simulink model "Basic_models_vfinal"  (R2019b)
settings: Solver=ode4  StartTime=0.0  StopTime=0.2  FixedStep=1e-5  MaxStep=1e-4  RelTol=1e-5
undefined symbols (not defined in the file or in its folder): C, L, R, R1
libraries: powerlib x82, powerlib_meascontrol x25
settings Model: Creator=eprie  LastModifiedBy=Edu Prieto

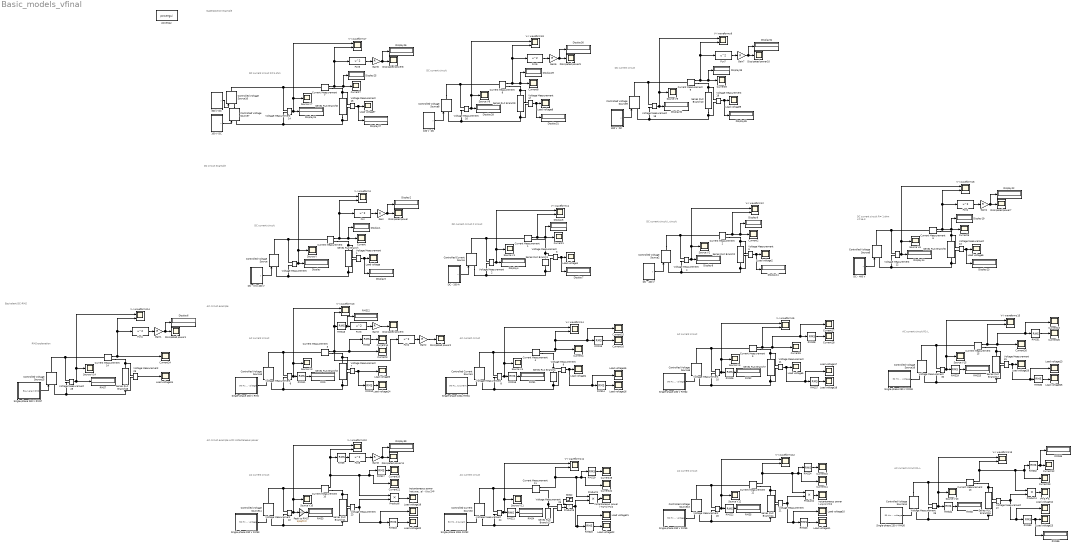
== system Basic_models_vfinal ==
  note: DC circuit example
  note: DC current circuit
  note: DC current circuit
      | C circuit
  note: DC current circuit
      | L circuit
  note: AC current circuit
  note: AC current circuit
  note: AC current circuit
  note: DC current circuit
      | R= 1 ohm L=1e-3
  note: DC current circuit
      | R=1 ohm
  note: DC current circuit
  note: DC current circuit
  note: Superposition example
  note: AC circuit example
  note: AC current circuit
  note: AC current circuit
  note: AC current circuit
  note: AC circuit example
      | with instantaneous power
  note: AC current circuit
      | R1-L
  note: RMS explanation
  note: Equivalent DC-RMS
  note: AC current circuit
      | R1-L
  "100 V  DC " : Subsystem
  100 V DC : Subsystem
  300 V  DC : Subsystem
  300 V DC : Subsystem
  Controlled Current Source : powerlib/Electrical Sources/Controlled Current Source  Initialize=on  Source_Type=AC  Amplitude=0  Phase=0  Frequency=0  Measurements=None
      settings: SourceProductName=Simscape Electrical
  Controlled Current Source1 : powerlib/Electrical Sources/Controlled Current Source  Initialize=off  Source_Type=AC  Amplitude=0  Phase=0  Frequency=0  Measurements=None
      settings: SourceProductName=Simscape Electrical
  Controlled Current Source2 : powerlib/Electrical Sources/Controlled Current Source  Initialize=off  Source_Type=AC  Amplitude=0  Phase=0  Frequency=0  Measurements=None
      settings: SourceProductName=Simscape Electrical
  Controlled Voltage Source{,2..3,5..11,13..16} (14 alike) : powerlib/Electrical Sources/Controlled Voltage Source  Initialize=on  Source_Type=AC  Amplitude=0  Phase=0  Frequency=0  Measurements=None
      settings: SourceProductName=Simscape Electrical
  Current{,1..26} (27 alike) : Scope
  Current Measurement{,1..15} (16 alike) : powerlib/Measurements/Current Measurement  PhasorSimulation=off  OutputType=Complex  PSBequivalent=0
      settings: SourceProductName=Simscape Electrical
  DC - 0 to 400 V : Subsystem
  DC - 200 A : Subsystem
  DC - 400 V : Subsystem
  "DC - 400 V  " : Subsystem
  Display{,1..9,11,14,19,22..35,39} (28 alike) : Display
  Dissipated power{,1..3,7..11} (9 alike) : Scope
  Fcn{,1..8} (9 alike) : Fcn  Expr=u^2
  Gain{,1..8} (9 alike) : Gain  Gain=R
  "Instantaneous power (+S/-S) P=0 " : Scope
  "Instantaneous power (+S/-S) P=0 " : Scope
  Instantaneous power (not average) - 0 to 2*P : Scope
  Load voltage{,1..26} (27 alike) : Scope
  P+S P-S : Scope
  Peak to RMS7 : Gain  Gain=1/sqrt(2)
  Product{1..2,4..6} (5 alike) : Product
  RMS{,1..7,12,25,35..36} (12 alike) : Display
  RMS{8..11,13..24,26..34} (25 alike) : powerlib_meascontrol/Measurements/RMS  TrueRMS=on  Freq=50  RMSInit=120  Ts=0
      settings: SourceProductName=Simscape Electrical
  Series RLC Branch{,3,8..11,16} (7 alike) : powerlib/Elements/Series RLC Branch  LConnTagsString=__new0  RConnTagsString=__new0  BranchType=R  Resistance=R  Inductance=1e-3  SetiL0=off  InitialCurrent=0  Capacitance=1e-6  Setx0=off  InitialVoltage=0  Measurements=None
      settings: SourceProductName=Simscape Electrical
  Series RLC Branch1 : powerlib/Elements/Series RLC Branch  LConnTagsString=__new0  RConnTagsString=__new0  BranchType=C  Resistance=R  Inductance=1e-3  SetiL0=off  InitialCurrent=0  Capacitance=C  Setx0=off  InitialVoltage=0  Measurements=None
      settings: SourceProductName=Simscape Electrical
  Series RLC Branch12 : powerlib/Elements/Series RLC Branch  LConnTagsString=__new0  RConnTagsString=__new0  BranchType=C  Resistance=1e-4  Inductance=1e-3  SetiL0=off  InitialCurrent=0  Capacitance=C  Setx0=off  InitialVoltage=400/sqrt(3)*sqrt(2)  Measurements=None
      settings: SourceProductName=Simscape Electrical
  Series RLC Branch14 : powerlib/Elements/Series RLC Branch  LConnTagsString=__new0  RConnTagsString=__new0  BranchType=L  Resistance=R  Inductance=L  SetiL0=off  InitialCurrent=0  Capacitance=1e-6  Setx0=off  InitialVoltage=0  Measurements=None
      settings: SourceProductName=Simscape Electrical
  Series RLC Branch15 : powerlib/Elements/Series RLC Branch  LConnTagsString=__new0  RConnTagsString=__new0  BranchType=RL  Resistance=R1  Inductance=L  SetiL0=off  InitialCurrent=0  Capacitance=1e-6  Setx0=off  InitialVoltage=0  Measurements=None
      settings: SourceProductName=Simscape Electrical
  Series RLC Branch17 : powerlib/Elements/Series RLC Branch  LConnTagsString=__new0  RConnTagsString=__new0  BranchType=RL  Resistance=R1  Inductance=L  SetiL0=off  InitialCurrent=0  Capacitance=1e-6  Setx0=off  InitialVoltage=0  Measurements=None
      settings: SourceProductName=Simscape Electrical
  Series RLC Branch2 : powerlib/Elements/Series RLC Branch  LConnTagsString=__new0  RConnTagsString=__new0  BranchType=L  Resistance=0.00001  Inductance=L  SetiL0=off  InitialCurrent=0  Capacitance=C  Setx0=off  InitialVoltage=0  Measurements=None
      settings: SourceProductName=Simscape Electrical
  Series RLC Branch4 : powerlib/Elements/Series RLC Branch  LConnTagsString=__new0  RConnTagsString=__new0  BranchType=C  Resistance=1e-4  Inductance=1e-3  SetiL0=off  InitialCurrent=0  Capacitance=C  Setx0=off  InitialVoltage=400/sqrt(3)*sqrt(2)  Measurements=None
      settings: SourceProductName=Simscape Electrical
  Series RLC Branch5 : powerlib/Elements/Series RLC Branch  LConnTagsString=__new0  RConnTagsString=__new0  BranchType=RL  Resistance=R  Inductance=L  SetiL0=off  InitialCurrent=0  Capacitance=1e-6  Setx0=off  InitialVoltage=0  Measurements=None
      settings: SourceProductName=Simscape Electrical
  Series RLC Branch7 : powerlib/Elements/Series RLC Branch  LConnTagsString=__new0  RConnTagsString=__new0  BranchType=L  Resistance=R  Inductance=L  SetiL0=off  InitialCurrent=0  Capacitance=1e-6  Setx0=off  InitialVoltage=0  Measurements=None
      settings: SourceProductName=Simscape Electrical
  Single-phase 100A RMS1 : Subsystem
  Single-phase 100A RMS2 : Subsystem
  Single-phase 230 V RMS : Subsystem
  Single-phase 230 V RMS2 : Subsystem
  Single-phase 230 V RMS3 : Subsystem
  Single-phase 230 V RMS5 : Subsystem
  Single-phase 230 V RMS6 : Subsystem
  Single-phase 230 V RMS7 : Subsystem
  Single-phase 230 V RMS8 : Subsystem
  Source V{,1..15} (16 alike) : Scope
  Step2 : Step  Time=0.01  SampleTime=0
  V-I waveforms{,1..15} (16 alike) : Scope  NumInputPorts=2
  Voltage Measurement{,1..31} (32 alike) : powerlib/Measurements/Voltage Measurement  PhasorSimulation=off  OutputType=Complex  PSBequivalent=0
      settings: SourceProductName=Simscape Electrical
  powergui : powerlib/powergui  Priority=1  SimulationMode=Discrete  SampleTime=1e-5  frequency=60  Iterations=50  frequencyindice=0  Pbase=100e6  ErrMax=1e-4  UnitsV=kV  UnitsW=MW  buscounter=0  FunctionMessages=off  echomessages=off  EnableUseOfTLC=off  CurrentSourceSwitches=off  DisableSnubberDevices=off  DisableRonSwitches=off  DisableVfSwitches=off  DisplayEquations=off  AutomaticDiscreteSolvers=off  SolverType=Tustin/Backward Euler (TBE)  Interpol=off  ExternalGateDelay=off  methode=off  Ts=100  x0status=blocks  SPID=on  SwTol=0  HookPort=off  NonlinearTolerance=1e-4  nMaxIteration=100  ContinueOnMaxIteration=off  RestoreLinks=warning  ResistiveCurrentMeasurement=off  Frange=[0:2:500]  Ylog=off  Xlog=on  ShowGrid=off  save=off  variable=ZData  structure=0  ZoomFFT=off  StartTime=0.0  cycles=1  DisplayStyle=1  fundamental=60  FreqAxis=off  MaxFrequency=1000  frequencyindicesteady=1  RmsSteady=1  display=off
      settings: SourceProductName=Simscape Electrical
  wires:
  Current Measurement/1 -> Current/1, Display1/1, V-I waveforms/2, Fcn/1
  DC - 0 to 400 V/1(v) -> Controlled Voltage Source/1
  Fcn/1 -> Gain/1
  Gain/1 -> Display2/1, Dissipated power/1
  Voltage Measurement/1 -> V-I waveforms/1, Source V/1, Display/1
  Voltage Measurement1/1 -> Display3/1, Load voltage/1
  Voltage Measurement3/1 -> Load voltage1/1, Display7/1
  Voltage Measurement2/1 -> Display4/1, Source V1/1, V-I waveforms1/1
  DC - 200 A/1(v) -> Controlled Current Source/1
  Current Measurement1/1 -> V-I waveforms1/2, Display5/1, Current1/1
  Current Measurement2/1 -> Current2/1, Display9/1, V-I waveforms2/2
  DC - 400 V/1(v) -> Controlled Voltage Source2/1
  Voltage Measurement4/1 -> V-I waveforms2/1, Source V2/1, Display8/1
  Voltage Measurement5/1 -> Display11/1, Load voltage2/1
  Voltage Measurement6/1 -> Source V3/1, V-I waveforms3/1, RMS11/1
  Gain3/1 -> Dissipated power3/1
  Fcn3/1 -> Gain3/1
  Single-phase 230 V RMS/1(50 Hz AC voltage) -> Controlled Voltage Source3/1
  RMS11/1 -> RMS/1
  RMS13/1 -> RMS12/1, Fcn3/1
  Voltage Measurement7/1 -> RMS10/1, Load voltage3/1
  Current Measurement3/1 -> RMS13/1, V-I waveforms3/2, Fcn2/1, RMS8/1, Current3/1
  Current Measurement4/1 -> V-I waveforms4/2, Current15/1, RMS15/1, Current4/1
  Voltage Measurement9/1 -> Load voltage15/1, RMS14/1, Load voltage4/1
  RMS16/1 -> RMS1/1
  Single-phase 100A RMS1/1(50 Hz AC current) -> Controlled Current Source1/1
  Voltage Measurement8/1 -> V-I waveforms4/1, Source V4/1, RMS16/1
  Voltage Measurement10/1 -> Source V5/1, V-I waveforms5/1, RMS26/1
  Single-phase 230 V RMS2/1(50 Hz AC voltage) -> Controlled Voltage Source5/1
  RMS26/1 -> RMS2/1
  Voltage Measurement11/1 -> RMS27/1, Load voltage17/1, Load voltage5/1
  Current Measurement5/1 -> V-I waveforms5/2, RMS28/1, Current17/1, Current5/1
  RMS10/1 -> Load voltage14/1
  RMS15/1 -> Current16/1
  RMS14/1 -> Load voltage16/1
  RMS28/1 -> Current18/1
  RMS27/1 -> Load voltage18/1
  Voltage Measurement13/1 -> Load voltage6/1, Display23/1
  Voltage Measurement12/1 -> Display14/1, Source V6/1, V-I waveforms6/1
  Gain4/1 -> Dissipated power7/1, Display22/1
  Fcn4/1 -> Gain4/1
  "DC - 400 V  "/1(v) -> Controlled Voltage Source6/1
  Current Measurement6/1 -> Fcn4/1, V-I waveforms6/2, Display19/1, Current6/1
  Voltage Measurement15/1 -> Load voltage7/1, Display27/1
  Voltage Measurement14/1 -> Display24/1, Source V7/1, V-I waveforms7/1
  Gain5/1 -> Dissipated power8/1, Display26/1
  Fcn5/1 -> Gain5/1
  100 V DC/1(v) -> Controlled Voltage Source7/1
  Current Measurement7/1 -> Fcn5/1, V-I waveforms7/2, Display25/1, Current7/1
  Current Measurement8/1 -> Current8/1, Display29/1, V-I waveforms8/2, Fcn6/1
  "100 V  DC "/1(v) -> Controlled Voltage Source8/1
  Fcn6/1 -> Gain6/1
  Gain6/1 -> Display30/1, Dissipated power9/1
  Voltage Measurement16/1 -> V-I waveforms8/1, Source V8/1, Display28/1
  Voltage Measurement17/1 -> Display31/1, Load voltage8/1
  Voltage Measurement19/1 -> Load voltage9/1, Display35/1
  Voltage Measurement18/1 -> Display32/1, Source V9/1, V-I waveforms9/1
  Gain7/1 -> Dissipated power10/1, Display34/1
  Fcn7/1 -> Gain7/1
  300 V  DC/1(v) -> Controlled Voltage Source9/1
  Current Measurement9/1 -> Fcn7/1, V-I waveforms9/2, Display33/1, Current9/1
  300 V DC/1(v) -> Controlled Voltage Source10/1
  RMS17/1 -> Current20/1
  Product6/1 -> Instantaneous power (not average) - 0 to 2*P/1
  RMS22/1 -> RMS5/1
  Single-phase 230 V RMS5/1(50 Hz AC voltage) -> Controlled Voltage Source13/1
  Voltage Measurement20/1 -> V-I waveforms12/1, Source V12/1, RMS22/1
  Voltage Measurement24/1 -> Source V11/1, V-I waveforms11/1, RMS21/1
  Single-phase 100A RMS2/1(50 Hz AC current) -> Controlled Current Source2/1
  RMS21/1 -> RMS4/1
  RMS9/1 -> Fcn8/1
  Peak to RMS7/1 -> RMS3/1
  Single-phase 230 V RMS3/1(50 Hz AC voltage) -> Controlled Voltage Source11/1
  Fcn8/1 -> Gain8/1
  Gain8/1 -> Display39/1, Dissipated power11/1
  Voltage Measurement22/1 -> V-I waveforms10/1, Source V10/1, Peak to RMS7/1
  Voltage Measurement26/1 -> RMS34/1, Source V13/1, V-I waveforms13/1
  Single-phase 230 V RMS6/1(50 Hz AC voltage) -> Controlled Voltage Source14/1
  RMS34/1 -> RMS6/1
  RMS8/1 -> Current14/1
  RMS18/1 -> Load voltage20/1
  Product5/1 -> Product1/2, RMS20/1, Load voltage21/1
  RMS20/1 -> Load voltage22/1
  Current Measurement11/1 -> Product1/1, Current22/1, RMS19/1, V-I waveforms11/2
  Product1/1 -> "Instantaneous power (+S/-S) P=0 "/1
  RMS19/1 -> Current19/1
  RMS24/1 -> Current10/1
  Product2/1 -> "Instantaneous power (+S/-S) P=0 "/1
  Current Measurement12/1 -> Current11/1, RMS24/1, Product2/1, V-I waveforms12/2
  RMS23/1 -> Load voltage11/1
  Voltage Measurement21/1 -> Product2/2, RMS23/1, Load voltage10/1
  Voltage Measurement27/1 -> Product4/2, RMS33/1, Load voltage12/1
  RMS33/1 -> RMS36/1, Load voltage23/1
  Current Measurement13/1 -> V-I waveforms13/2, Product4/1, RMS32/1, Current23/1
  Product4/1 -> P+S P-S/1
  RMS32/1 -> RMS35/1, Current12/1
  Current Measurement10/1 -> Product6/1, Current21/1, RMS17/1, RMS9/1, V-I waveforms10/2
  Voltage Measurement23/1 -> Product6/2, RMS18/1, Load voltage19/1
  Step2/1 -> Product5/1
  Voltage Measurement25/1 -> Product5/2
  Voltage Measurement29/1 -> Load voltage24/1
  Current Measurement14/1 -> Current24/1, Fcn1/1, V-I waveforms14/2
  Voltage Measurement28/1 -> RMS7/1, V-I waveforms14/1, Source V14/1
  Single-phase 230 V RMS7/1(Equivalent RMS) -> Controlled Voltage Source15/1
  Fcn1/1 -> Gain1/1
  Gain1/1 -> Display6/1, Dissipated power1/1
  RMS30/1 -> Load voltage25/1
  RMS31/1 -> Current25/1
  Current Measurement15/1 -> Current26/1, RMS31/1, Current13/1, V-I waveforms15/2
  Voltage Measurement31/1 -> Load voltage26/1, Load voltage13/1, RMS30/1
  RMS29/1 -> RMS25/1
  Single-phase 230 V RMS8/1(50 Hz AC voltage) -> Controlled Voltage Source16/1
  Voltage Measurement30/1 -> V-I waveforms15/1, Source V15/1, RMS29/1
  Fcn2/1 -> Gain2/1
  Gain2/1 -> Dissipated power2/1
  connections:
  Current Measurement/LConn1 -- Voltage Measurement/LConn1 -- Controlled Voltage Source/RConn1
  Current Measurement/RConn1 -- Series RLC Branch/LConn1 -- Voltage Measurement1/LConn1
  Series RLC Branch/RConn1 -- Voltage Measurement/LConn2 -- Controlled Voltage Source/LConn1 -- Voltage Measurement1/LConn2
  Voltage Measurement2/LConn1 -- Controlled Current Source/RConn1 -- Current Measurement1/LConn1
  Series RLC Branch1/RConn1 -- Voltage Measurement3/LConn2 -- Controlled Current Source/LConn1 -- Voltage Measurement2/LConn2
  Controlled Voltage Source2/RConn1 -- Voltage Measurement4/LConn1 -- Current Measurement2/LConn1
  Voltage Measurement5/LConn1 -- Current Measurement2/RConn1 -- Series RLC Branch2/LConn1
  Voltage Measurement5/LConn2 -- Series RLC Branch2/RConn1 -- Voltage Measurement4/LConn2 -- Controlled Voltage Source2/LConn1
  Voltage Measurement6/LConn1 -- Current Measurement3/LConn1 -- Controlled Voltage Source3/RConn1
  Current Measurement3/RConn1 -- Voltage Measurement7/LConn1 -- Series RLC Branch3/LConn1
  Series RLC Branch3/RConn1 -- Voltage Measurement7/LConn2 -- Voltage Measurement6/LConn2 -- Controlled Voltage Source3/LConn1
  Voltage Measurement8/LConn1 -- Controlled Current Source1/RConn1 -- Current Measurement4/LConn1
  Controlled Current Source1/LConn1 -- Voltage Measurement8/LConn2 -- Series RLC Branch4/RConn1 -- Voltage Measurement9/LConn2
  Voltage Measurement10/LConn1 -- Current Measurement5/LConn1 -- Controlled Voltage Source5/RConn1
  Current Measurement5/RConn1 -- Voltage Measurement11/LConn1 -- Series RLC Branch7/LConn1
  Voltage Measurement10/LConn2 -- Series RLC Branch7/RConn1 -- Voltage Measurement11/LConn2 -- Controlled Voltage Source5/LConn1
  Voltage Measurement9/LConn1 -- Current Measurement4/RConn1 -- Series RLC Branch4/LConn1
  Current Measurement6/LConn1 -- Voltage Measurement12/LConn1 -- Controlled Voltage Source6/RConn1
  Current Measurement6/RConn1 -- Voltage Measurement13/LConn1 -- Series RLC Branch5/LConn1
  Series RLC Branch5/RConn1 -- Voltage Measurement13/LConn2 -- Voltage Measurement12/LConn2 -- Controlled Voltage Source6/LConn1
  Current Measurement7/LConn1 -- Controlled Voltage Source10/RConn1 -- Voltage Measurement14/LConn1
  Current Measurement7/RConn1 -- Voltage Measurement15/LConn1 -- Series RLC Branch8/LConn1
  Series RLC Branch8/RConn1 -- Voltage Measurement15/LConn2 -- Voltage Measurement14/LConn2 -- Controlled Voltage Source7/LConn1
  Controlled Voltage Source8/RConn1 -- Current Measurement8/LConn1 -- Voltage Measurement16/LConn1
  Voltage Measurement17/LConn1 -- Current Measurement8/RConn1 -- Series RLC Branch9/LConn1
  Controlled Voltage Source8/LConn1 -- Series RLC Branch9/RConn1 -- Voltage Measurement17/LConn2 -- Voltage Measurement16/LConn2
  Current Measurement9/LConn1 -- Voltage Measurement18/LConn1 -- Controlled Voltage Source9/RConn1
  Current Measurement9/RConn1 -- Voltage Measurement19/LConn1 -- Series RLC Branch10/LConn1
  Series RLC Branch10/RConn1 -- Voltage Measurement18/LConn2 -- Controlled Voltage Source9/LConn1 -- Voltage Measurement19/LConn2
  Controlled Voltage Source10/LConn1 -- Controlled Voltage Source7/RConn1
  Voltage Measurement22/LConn1 -- Controlled Voltage Source11/RConn1 -- Current Measurement10/LConn1
  Current Measurement10/RConn1 -- Series RLC Branch11/LConn1 -- Voltage Measurement23/LConn1
  Series RLC Branch11/RConn1 -- Controlled Voltage Source11/LConn1 -- Voltage Measurement22/LConn2 -- Voltage Measurement23/LConn2
  Voltage Measurement24/LConn1 -- Controlled Current Source2/RConn1 -- Current Measurement11/LConn1
  Voltage Measurement24/LConn2 -- Controlled Current Source2/LConn1 -- Series RLC Branch12/RConn1 -- Voltage Measurement25/LConn2
  Voltage Measurement20/LConn1 -- Controlled Voltage Source13/RConn1 -- Current Measurement12/LConn1
  Current Measurement12/RConn1 -- Series RLC Branch14/LConn1 -- Voltage Measurement21/LConn1
  Voltage Measurement20/LConn2 -- Controlled Voltage Source13/LConn1 -- Voltage Measurement21/LConn2 -- Series RLC Branch14/RConn1
  Voltage Measurement25/LConn1 -- Current Measurement11/RConn1 -- Series RLC Branch12/LConn1
  Controlled Voltage Source14/RConn1 -- Voltage Measurement26/LConn1 -- Current Measurement13/LConn1
  Series RLC Branch15/LConn1 -- Current Measurement13/RConn1 -- Voltage Measurement27/LConn1
  Voltage Measurement27/LConn2 -- Voltage Measurement26/LConn2 -- Controlled Voltage Source14/LConn1 -- Series RLC Branch15/RConn1
  Voltage Measurement28/LConn1 -- Controlled Voltage Source15/RConn1 -- Current Measurement14/LConn1
  Current Measurement14/RConn1 -- Series RLC Branch16/LConn1 -- Voltage Measurement29/LConn1
  Series RLC Branch16/RConn1 -- Controlled Voltage Source15/LConn1 -- Voltage Measurement28/LConn2 -- Voltage Measurement29/LConn2
  Voltage Measurement30/LConn1 -- Controlled Voltage Source16/RConn1 -- Current Measurement15/LConn1
  Current Measurement15/RConn1 -- Series RLC Branch17/LConn1 -- Voltage Measurement31/LConn1
  Voltage Measurement30/LConn2 -- Controlled Voltage Source16/LConn1 -- Voltage Measurement31/LConn2 -- Series RLC Branch17/RConn1
  Voltage Measurement3/LConn1 -- Series RLC Branch1/LConn1 -- Current Measurement1/RConn1

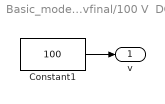
== system Basic_models_vfinal/100 V  DC  ==
  Constant1 : Constant  Value=100
  v : Outport
  wires:
  Constant1/1 -> v/1

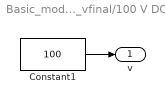
== system Basic_models_vfinal/100 V DC ==
  Constant1 : Constant  Value=100
  v : Outport
  wires:
  Constant1/1 -> v/1

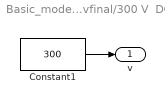
== system Basic_models_vfinal/300 V  DC ==
  Constant1 : Constant  Value=300
  v : Outport
  wires:
  Constant1/1 -> v/1

== system Basic_models_vfinal/300 V DC ==
  Constant1 : Constant  Value=300
  v : Outport
  wires:
  Constant1/1 -> v/1

== system Basic_models_vfinal/DC - 0 to 400 V ==
  Constant1 : Constant  Value=400
  v : Outport
  wires:
  Constant1/1 -> v/1

== system Basic_models_vfinal/DC - 200 A ==
  Constant1 : Constant  Value=400
  v : Outport
  wires:
  Constant1/1 -> v/1

== system Basic_models_vfinal/DC - 400 V ==
  Constant1 : Constant  Value=400
  v : Outport
  wires:
  Constant1/1 -> v/1

== system Basic_models_vfinal/DC - 400 V   ==
  Constant1 : Constant  Value=400
  v : Outport
  wires:
  Constant1/1 -> v/1

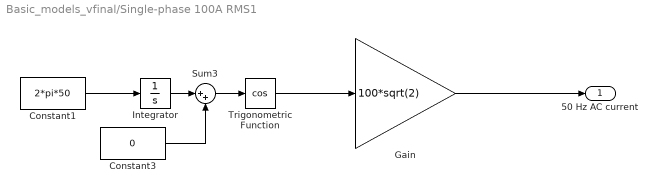
== system Basic_models_vfinal/Single-phase 100A RMS1 ==
  Constant1 : Constant  Value=2*pi*50
  Constant3 : Constant  Value=0
  Gain : Gain  Gain=100*sqrt(2)
  Integrator : Integrator
  Sum3 : Sum  Inputs=|++
  Trigonometric Function : Trigonometry  Operator=cos
  50 Hz AC current : Outport
  wires:
  Gain/1 -> 50 Hz AC current/1
  Trigonometric Function/1 -> Gain/1
  Integrator/1 -> Sum3/1
  Constant1/1 -> Integrator/1
  Sum3/1 -> Trigonometric Function/1
  Constant3/1 -> Sum3/2

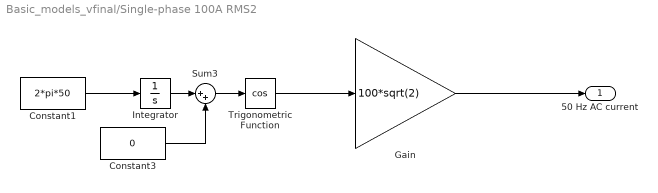
== system Basic_models_vfinal/Single-phase 100A RMS2 ==
  Constant1 : Constant  Value=2*pi*50
  Constant3 : Constant  Value=0
  Gain : Gain  Gain=100*sqrt(2)
  Integrator : Integrator
  Sum3 : Sum  Inputs=|++
  Trigonometric Function : Trigonometry  Operator=cos
  50 Hz AC current : Outport
  wires:
  Constant3/1 -> Sum3/2
  Sum3/1 -> Trigonometric Function/1
  Constant1/1 -> Integrator/1
  Integrator/1 -> Sum3/1
  Trigonometric Function/1 -> Gain/1
  Gain/1 -> 50 Hz AC current/1

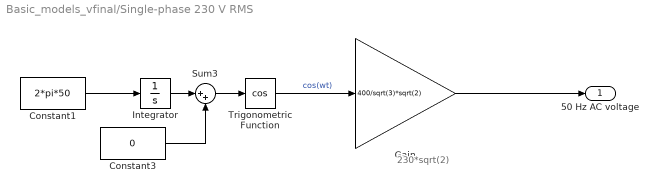
== system Basic_models_vfinal/Single-phase 230 V RMS ==
  note: 230*sqrt(2)
  Constant1 : Constant  Value=2*pi*50
  Constant3 : Constant  Value=0
  Gain : Gain  Gain=400/sqrt(3)*sqrt(2)
  Integrator : Integrator
  Sum3 : Sum  Inputs=|++
  Trigonometric Function : Trigonometry  Operator=cos
  50 Hz AC voltage : Outport
  wires:
  Constant3/1 -> Sum3/2
  Sum3/1 -> Trigonometric Function/1
  Constant1/1 -> Integrator/1
  Integrator/1 -> Sum3/1
  Trigonometric Function/1 -> Gain/1  "cos(wt)"
  Gain/1 -> 50 Hz AC voltage/1

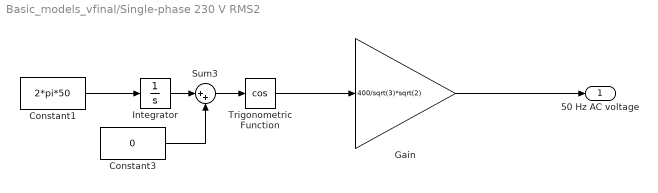
== system Basic_models_vfinal/Single-phase 230 V RMS2 ==
  Constant1 : Constant  Value=2*pi*50
  Constant3 : Constant  Value=0
  Gain : Gain  Gain=400/sqrt(3)*sqrt(2)
  Integrator : Integrator
  Sum3 : Sum  Inputs=|++
  Trigonometric Function : Trigonometry  Operator=cos
  50 Hz AC voltage : Outport
  wires:
  Constant3/1 -> Sum3/2
  Sum3/1 -> Trigonometric Function/1
  Constant1/1 -> Integrator/1
  Integrator/1 -> Sum3/1
  Trigonometric Function/1 -> Gain/1
  Gain/1 -> 50 Hz AC voltage/1

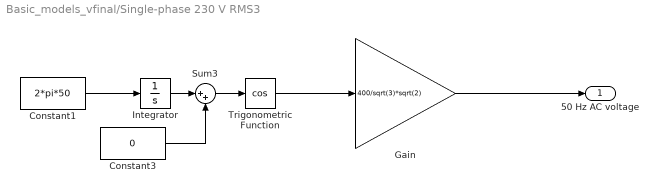
== system Basic_models_vfinal/Single-phase 230 V RMS3 ==
  Constant1 : Constant  Value=2*pi*50
  Constant3 : Constant  Value=0
  Gain : Gain  Gain=400/sqrt(3)*sqrt(2)
  Integrator : Integrator
  Sum3 : Sum  Inputs=|++
  Trigonometric Function : Trigonometry  Operator=cos
  50 Hz AC voltage : Outport
  wires:
  Gain/1 -> 50 Hz AC voltage/1
  Trigonometric Function/1 -> Gain/1
  Integrator/1 -> Sum3/1
  Constant1/1 -> Integrator/1
  Sum3/1 -> Trigonometric Function/1
  Constant3/1 -> Sum3/2

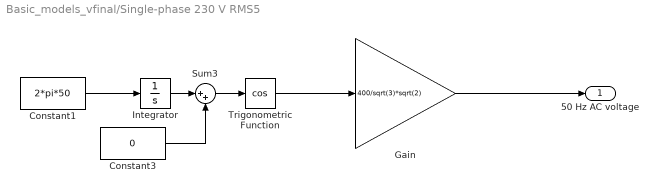
== system Basic_models_vfinal/Single-phase 230 V RMS5 ==
  Constant1 : Constant  Value=2*pi*50
  Constant3 : Constant  Value=0
  Gain : Gain  Gain=400/sqrt(3)*sqrt(2)
  Integrator : Integrator
  Sum3 : Sum  Inputs=|++
  Trigonometric Function : Trigonometry  Operator=cos
  50 Hz AC voltage : Outport
  wires:
  Gain/1 -> 50 Hz AC voltage/1
  Trigonometric Function/1 -> Gain/1
  Integrator/1 -> Sum3/1
  Constant1/1 -> Integrator/1
  Sum3/1 -> Trigonometric Function/1
  Constant3/1 -> Sum3/2

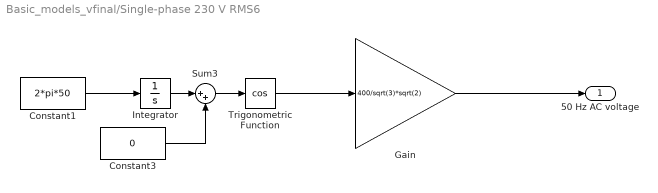
== system Basic_models_vfinal/Single-phase 230 V RMS6 ==
  Constant1 : Constant  Value=2*pi*50
  Constant3 : Constant  Value=0
  Gain : Gain  Gain=400/sqrt(3)*sqrt(2)
  Integrator : Integrator
  Sum3 : Sum  Inputs=|++
  Trigonometric Function : Trigonometry  Operator=cos
  50 Hz AC voltage : Outport
  wires:
  Constant3/1 -> Sum3/2
  Sum3/1 -> Trigonometric Function/1
  Constant1/1 -> Integrator/1
  Integrator/1 -> Sum3/1
  Trigonometric Function/1 -> Gain/1
  Gain/1 -> 50 Hz AC voltage/1

== system Basic_models_vfinal/Single-phase 230 V RMS7 ==
  Constant1 : Constant  Value=400/sqrt(3)
  Equivalent RMS : Outport
  wires:
  Constant1/1 -> Equivalent RMS/1

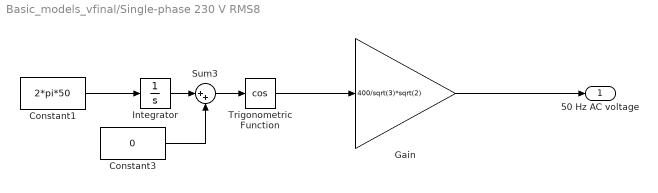
== system Basic_models_vfinal/Single-phase 230 V RMS8 ==
  Constant1 : Constant  Value=2*pi*50
  Constant3 : Constant  Value=0
  Gain : Gain  Gain=400/sqrt(3)*sqrt(2)
  Integrator : Integrator
  Sum3 : Sum  Inputs=|++
  Trigonometric Function : Trigonometry  Operator=cos
  50 Hz AC voltage : Outport
  wires:
  Gain/1 -> 50 Hz AC voltage/1
  Trigonometric Function/1 -> Gain/1
  Integrator/1 -> Sum3/1
  Constant1/1 -> Integrator/1
  Sum3/1 -> Trigonometric Function/1
  Constant3/1 -> Sum3/2
